simulink model "Model_kyvadla_na_voziku_m_slx"  (R2020a)
settings: Solver=FixedStepAuto  StartTime=0.0  StopTime=50  FixedStep=0.01  RelTol=1e-3
values from neighbouring files (symbols this model uses):
  dphi = 0    [Model_kyvadla_na_voziku_m.m]
  dx = 0    [Model_kyvadla_na_voziku_m.m]
  f = 100    [Model_kyvadla_na_voziku_m.m]
  g = 9.81    [Model_kyvadla_na_voziku_m.m]
  l = 1    [Model_kyvadla_na_voziku_m.m]
  m = 10    [Model_kyvadla_na_voziku_m.m]
  M = 50    [Model_kyvadla_na_voziku_m.m]
  phi = 20    [Model_kyvadla_na_voziku_m.m]
  x = 0    [Model_kyvadla_na_voziku_m.m]
settings Model: Creator=Jiří  LastModifiedBy=Jiří

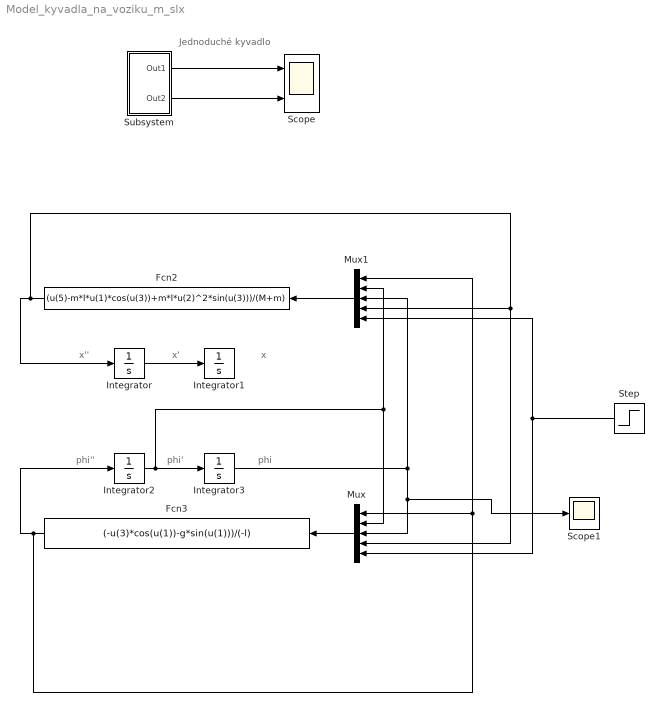
== system Model_kyvadla_na_voziku_m_slx ==
  note: phi
  note: phi''
  note: phi'
  note: x
  note: x'
  note: x''
  note: Jednoduché kyvadlo
  Fcn2 : Fcn  Expr=(u(5)-m*l*u(1)*cos(u(3))+m*l*u(2)^2*sin(u(3)))/(M+m)
  Fcn3 : Fcn  Expr=(-u(3)*cos(u(1))-g*sin(u(1)))/(-l)
  Integrator : Integrator  InitialCondition=dx
  Integrator1 : Integrator  InitialCondition=x
  Integrator2 : Integrator  InitialCondition=dphi
  Integrator3 : Integrator  InitialCondition=phi
  Mux : Mux  Inputs=5
  Mux1 : Mux  Inputs=5
  Scope : Scope  NumInputPorts=2
  Scope1 : Scope
  Step : Step  Time=5  After=f  SampleTime=1
  Subsystem : Subsystem
  wires:
  Subsystem/1(Out1) -> Scope/1
  Subsystem/2(Out2) -> Scope/2
  Integrator2/1 -> Mux/2, Mux1/2, Integrator3/1
  Mux/1 -> Fcn3/1
  Integrator/1 -> Integrator1/1
  Fcn2/1 -> Mux1/4, Mux/4, Integrator/1
  Fcn3/1 -> Mux1/1, Mux/1, Integrator2/1
  Mux1/1 -> Fcn2/1
  Integrator3/1 -> Scope1/1, Mux/3, Mux1/3
  Step/1 -> Mux1/5, Mux/5

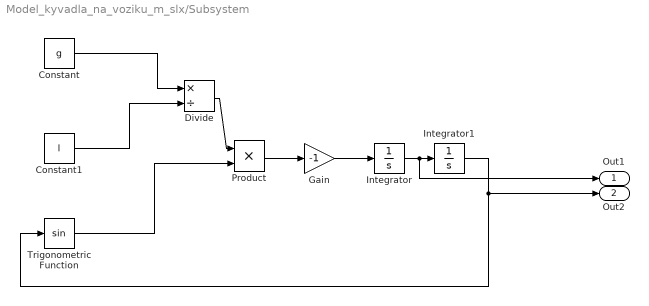
== system Model_kyvadla_na_voziku_m_slx/Subsystem ==
  Constant : Constant  Value=g
  Constant1 : Constant  Value=l
  Divide : Product  Inputs=*/
  Gain : Gain  Gain=-1
  Integrator : Integrator
  Integrator1 : Integrator  InitialCondition=1
  Product : Product
  Trigonometric Function : Trigonometry
  Out1 : Outport
  Out2 : Outport  Port=2
  wires:
  Gain/1 -> Integrator/1
  Integrator/1 -> Out1/1, Integrator1/1
  Constant/1 -> Divide/1
  Trigonometric Function/1 -> Product/2
  Divide/1 -> Product/1
  Product/1 -> Gain/1
  Constant1/1 -> Divide/2
  Integrator1/1 -> Out2/1, Trigonometric Function/1
